simulink model "corBO3"  (R2016b)
settings: Solver=VariableStepAuto  StartTime=0.0  StopTime=2  RelTol=1e-3
values from neighbouring files (symbols this model uses):
  Ki = 43.2/1000    (= 0.0432)    [Cons.m]
  Kred = 35.9    [Cons.m]
  meq = 120    [Cons.m]
  rpignon = 21*0.8/(2*1000)    (= 0.0084)    [Cons.m]
settings Model: Creator=emiliendurif  LastModifiedBy=emiliendurif

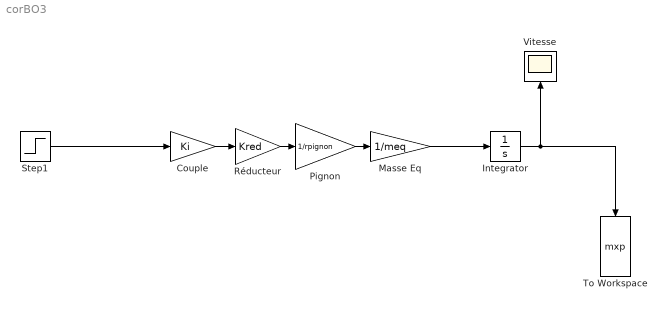
== system corBO3 ==
  Couple : Gain  Gain=Ki
  Integrator : Integrator
  Masse Eq : Gain  Gain=1/meq
  Pignon : Gain  Gain=1/rpignon
  Réducteur : Gain  Gain=Kred
  Step1 : Step  Time=0.1  After=0.2  SampleTime=0
  To Workspace : ToWorkspace  VariableName=mxp  SaveFormat=Timeseries  SampleTime=-1
  Vitesse : Scope
  wires:
  Pignon/1 -> Masse Eq/1
  Integrator/1 -> To Workspace/1, Vitesse/1
  Masse Eq/1 -> Integrator/1
  Réducteur/1 -> Pignon/1
  Couple/1 -> Réducteur/1
  Step1/1 -> Couple/1
